simulink model "hw3s"  (Simulink 9.2)
settings: Solver=ode5  StartTime=0.0  StopTime=11  FixedStep=0.001  RelTol=1e-3
values from neighbouring files (symbols this model uses):
  a = 1.14    [hw3a.m]
  b = L-a    (= 1.4)    [hw3a.m]
  Cf = 44000*2    (= 88000)    [hw3a.m]
  Cr = 47000*2    (= 94000)    [hw3a.m]
  Iz = 2420.0    (= 2420)    [hw3a.m]
  KD = 1.2    [hw3a.m]
  KP = 1.2    [hw3a.m]
  m = 1500    [hw3a.m]
  x0 = x    [road_shape.m]
  y0 = y    [road_shape.m]
settings Model: Creator=Changsun Ahn  LastModifiedBy=Changsun Ahn
settings DataIOCC: SignalLoggingName=sigsOut
settings OptimizationCC: ExpressionDepthLimit=2147483647
settings DebuggingCC: SaveWithParameterizedLinksMsg=none  SignalResolutionControl=TryResolveAllWithWarning  MultiTaskDSMMsg=warning  MultiTaskCondExecSysMsg=none  FcnCallInpInsideContextMsg=error
settings HardwareCC: TargetBitPerPointer=64  TargetBitPerSizeT=64  TargetBitPerPtrDiffT=64  TargetLongLongMode=on  TargetIntDivRoundTo=Zero  TargetEndianess=LittleEndian  TargetWordSize=64  TargetHWDeviceType=MATLAB Host  ProdEqTarget=off

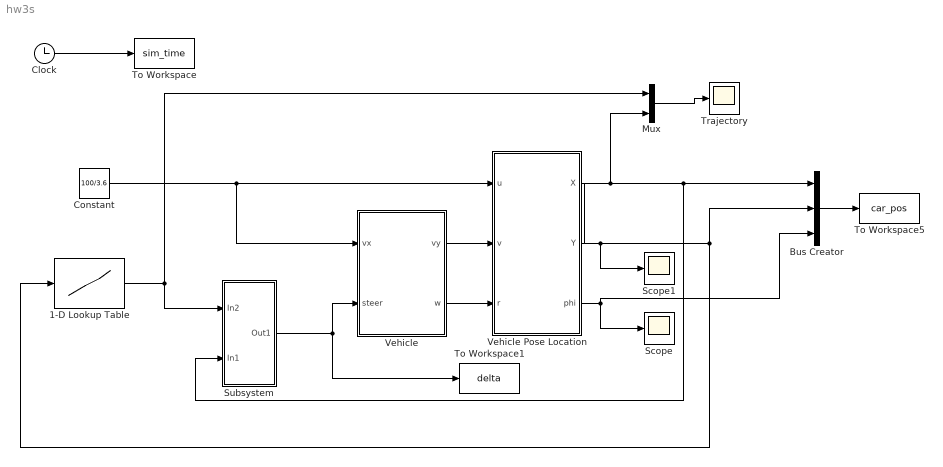
== system hw3s ==
  1-D Lookup Table : Lookup_n-D  NumberOfTableDimensions=1  BreakpointsForDimension1=x0  Table=y0  InternalRulePriority=Speed  RndMeth=Simplest  InputSameDT=on
  Bus Creator : BusCreator  Inputs=3
  Clock : Clock
  Constant : Constant  Value=100/3.6
  Mux : Mux  Inputs=2
  Scope : Scope
  Scope1 : Scope
  Subsystem : Subsystem
  To Workspace : ToWorkspace  VariableName=sim_time  SampleTime=-1
  To Workspace1 : ToWorkspace  VariableName=delta  SaveFormat=Timeseries  SampleTime=-1
  To Workspace5 : ToWorkspace  VariableName=car_pos  SaveFormat=Timeseries  SampleTime=-1
  Trajectory : Scope
  Vehicle : Subsystem
  Vehicle Pose Location : Subsystem
  wires:
  Vehicle/1(vy) -> Vehicle Pose Location/2(v)
  Vehicle/2(w) -> Vehicle Pose Location/3(r)
  Vehicle Pose Location/2(Y) -> Subsystem/2(In1), Bus Creator/1, Mux/2
  Vehicle Pose Location/3(phi) -> Bus Creator/3, Scope/1
  Vehicle Pose Location/1(X) -> Bus Creator/2, 1-D Lookup Table/1, Scope1/1
  Clock/1 -> To Workspace/1
  Constant/1 -> Vehicle/1(vx), Vehicle Pose Location/1(u)
  1-D Lookup Table/1 -> Subsystem/1(In2), Mux/1
  Mux/1 -> Trajectory/1
  Subsystem/1(Out1) -> To Workspace1/1, Vehicle/2(steer)
  Bus Creator/1 -> To Workspace5/1

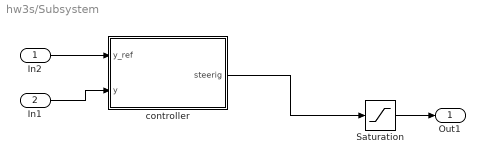
== system hw3s/Subsystem ==
  In2 : Inport
  In1 : Inport  Port=2
  Saturation : Saturate  UpperLimit=30*pi/180  LowerLimit=-30*pi/180
  controller : Subsystem
  Out1 : Outport
  wires:
  In1/1 -> controller/2(y)
  In2/1 -> controller/1(y_ref)
  Saturation/1 -> Out1/1
  controller/1(steerig) -> Saturation/1

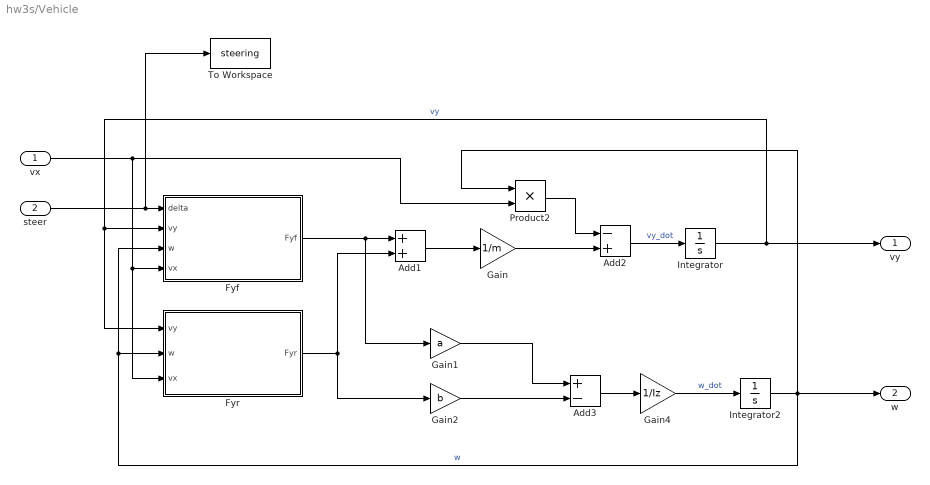
== system hw3s/Vehicle ==
  vx : Inport
  steer : Inport  Port=2
  Add1 : Sum
  Add2 : Sum  Inputs=-+
  Add3 : Sum  Inputs=+-
  Fyf : Subsystem
  Fyr : Subsystem
  Gain : Gain  Gain=1/m
  Gain1 : Gain  Gain=a
  Gain2 : Gain  Gain=b
  Gain4 : Gain  Gain=1/Iz
  Integrator : Integrator
  Integrator2 : Integrator
  Product2 : Product  RndMeth=Zero
  To Workspace : ToWorkspace  VariableName=steering  SaveFormat=Timeseries  SampleTime=-1
  vy : Outport
  w : Outport  Port=2
  wires:
  Add1/1 -> Gain/1
  Gain/1 -> Add2/2
  vx/1 -> Fyr/3(vx), Fyf/4(vx), Product2/2
  Product2/1 -> Add2/1
  Add2/1 -> Integrator/1  "vy_dot"
  Fyf/1(Fyf) -> Gain1/1, Add1/1
  Fyr/1(Fyr) -> Gain2/1, Add1/2
  Integrator/1 -> vy/1, Fyf/2(vy), Fyr/1(vy)  "vy"
  Gain1/1 -> Add3/1
  Gain2/1 -> Add3/2
  Add3/1 -> Gain4/1
  Gain4/1 -> Integrator2/1  "w_dot"
  Integrator2/1 -> w/1, Product2/1, Fyf/3(w), Fyr/2(w)  "w"
  steer/1 -> To Workspace/1, Fyf/1(delta)

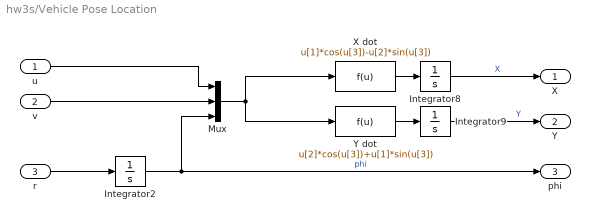
== system hw3s/Vehicle Pose Location ==
  u : Inport
  v : Inport  Port=2
  r : Inport  Port=3
  Integrator2 : Integrator
  Integrator8 : Integrator
  Integrator9 : Integrator
  Mux : Mux  Inputs=3
  X dot : Fcn  Expr=u[1]*cos(u[3])-u[2]*sin(u[3])
  Y dot : Fcn  Expr=u[2]*cos(u[3])+u[1]*sin(u[3])  SampleTime=0
  X : Outport
  Y : Outport  Port=2
  phi : Outport  Port=3
  wires:
  r/1 -> Integrator2/1
  Integrator2/1 -> phi/1, Mux/3  "phi"
  Mux/1 -> Y dot/1, X dot/1
  Y dot/1 -> Integrator9/1
  X dot/1 -> Integrator8/1
  Integrator9/1 -> Y/1  "Y"
  Integrator8/1 -> X/1  "X"
  v/1 -> Mux/2
  u/1 -> Mux/1

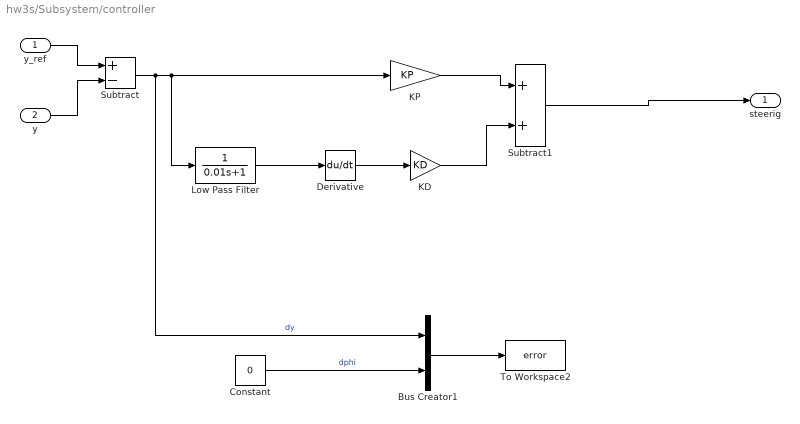
== system hw3s/Subsystem/controller ==
  y_ref : Inport
  y : Inport  Port=2
  Bus Creator1 : BusCreator  Inputs=2
  Constant : Constant  Value=0
  Derivative : Derivative
  KD : Gain  Gain=KD
  KP : Gain  Gain=KP
  Low Pass Filter : TransferFcn  Denominator=[0.01 1]
  Subtract : Sum  Inputs=+-
  Subtract1 : Sum
  To Workspace2 : ToWorkspace  VariableName=error  SaveFormat=Timeseries  SampleTime=-1
  steerig : Outport
  wires:
  y_ref/1 -> Subtract/1
  y/1 -> Subtract/2
  Subtract/1 -> Bus Creator1/1, Low Pass Filter/1, KP/1  "dy"
  Low Pass Filter/1 -> Derivative/1
  Derivative/1 -> KD/1
  KP/1 -> Subtract1/1
  KD/1 -> Subtract1/2
  Subtract1/1 -> steerig/1
  Bus Creator1/1 -> To Workspace2/1
  Constant/1 -> Bus Creator1/2  "dphi"

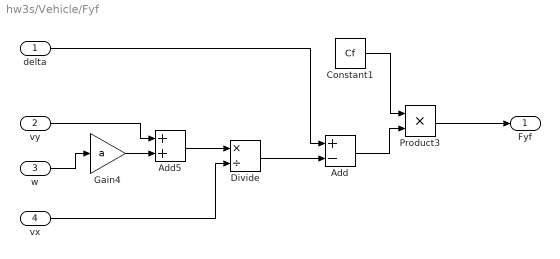
== system hw3s/Vehicle/Fyf ==
  delta : Inport
  vy : Inport  Port=2
  w : Inport  Port=3
  vx : Inport  Port=4
  Add : Sum  Inputs=+-
  Add5 : Sum
  Constant1 : Constant  Value=Cf
  Divide : Product  Inputs=*/
  Gain4 : Gain  Gain=a
  Product3 : Product  RndMeth=Zero
  Fyf : Outport
  wires:
  w/1 -> Gain4/1
  vy/1 -> Add5/1
  Add5/1 -> Divide/1
  Gain4/1 -> Add5/2
  vx/1 -> Divide/2
  Constant1/1 -> Product3/1
  Add/1 -> Product3/2
  Divide/1 -> Add/2
  delta/1 -> Add/1
  Product3/1 -> Fyf/1

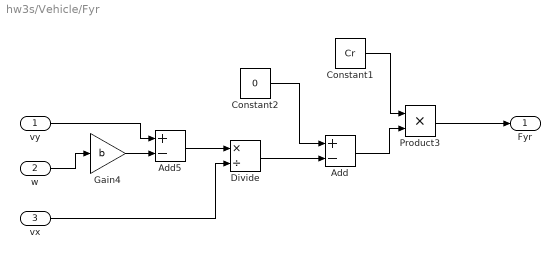
== system hw3s/Vehicle/Fyr ==
  vy : Inport
  w : Inport  Port=2
  vx : Inport  Port=3
  Add : Sum  Inputs=+-
  Add5 : Sum  Inputs=+-
  Constant1 : Constant  Value=Cr
  Constant2 : Constant  Value=0
  Divide : Product  Inputs=*/
  Gain4 : Gain  Gain=b
  Product3 : Product  RndMeth=Zero
  Fyr : Outport
  wires:
  w/1 -> Gain4/1
  vy/1 -> Add5/1
  Add5/1 -> Divide/1
  Gain4/1 -> Add5/2
  vx/1 -> Divide/2
  Constant1/1 -> Product3/1
  Add/1 -> Product3/2
  Divide/1 -> Add/2
  Product3/1 -> Fyr/1
  Constant2/1 -> Add/1
